simulink model "MORUS_NELINEARNI_NELINEARNI_YAW"  (R2019a)
settings: Solver=FixedStepAuto  StartTime=0.0  StopTime=sim_time  RelTol=1e-3  EnableMultiTasking=on
values from neighbouring files (symbols this model uses):
  A_dis_calc = expm(kSamplingTime*A_continous_time)    [MPC_designer_X.m]    (also in NonTilting.m; RUN_simulation.m; Simulacija_MPC_YAW_NELINEARNI.m; Simulacija_MPC_Z.m)
  A_dis_calc_YAW = expm(kSamplingTime_YAW*A_continous_time_YAW)    [Simulacija_MPC_YAW_NELINEARNI.m]
  B_dis_calc = integral_exp_A * B_continous_time    [MPC_designer_X.m]    (also in NonTilting.m; RUN_simulation.m; Simulacija_MPC_YAW_NELINEARNI.m; Simulacija_MPC_Z.m)
  B_dis_calc_YAW = integral_exp_A_YAW * B_continous_time_YAW    [Simulacija_MPC_YAW_NELINEARNI.m]
  b_f = 4.56e-4    (= 0.000456)    [LinearizacijaMatrica.m]    (also in Linearizirane_matrice.mat; MPC_designer_X.m; NonTilting.m; RUN_simulation.m)
  b_m = 0.01    [LinearizacijaMatrica.m]    (also in Linearizirane_matrice.mat; MPC_designer_X.m; NonTilting.m; RUN_simulation.m)
  BETA = 0.0    (= 0)    [LinearizacijaMatrica.m]    (also in Linearizirane_matrice.mat; MPC_designer_X.m; NonTilting.m = 0.200712863979; RUN_simulation.m)
  g = 9.80665    [LinearizacijaMatrica.m]    (also in Linearizirane_matrice.mat; MPC_designer_X.m = 9.81; NonTilting.m = 9.81; RUN_simulation.m = 9.81)
  hover = 427.6233    [MPC_designer_X.m]    (also in NonTilting.m; RUN_simulation.m; Simulacija_MPC_YAW_NELINEARNI.m; Simulacija_MPC_Z.m)
  I_b_xx = 5.5268    [MPC_designer_X.m]    (also in NonTilting.m; RUN_simulation.m; Simulacija_MPC_YAW_NELINEARNI.m; Simulacija_MPC_Z.m)
  I_b_yy = 5.5268    [MPC_designer_X.m]    (also in NonTilting.m; RUN_simulation.m; Simulacija_MPC_YAW_NELINEARNI.m; Simulacija_MPC_Z.m)
  I_b_zz = 6.8854    [MPC_designer_X.m]    (also in NonTilting.m; RUN_simulation.m; Simulacija_MPC_YAW_NELINEARNI.m; Simulacija_MPC_Z.m)
  kSamplingTime = 0.810    (= 0.81)    [MPCDesigner_YAW.m]    (also in MPC_designer_X.m = 0.1; MPC_designer_Z.m; NonTilting.m = 0.015; RUN_simulation.m = 0.015)
  kSamplingTime_YAW = 0.105    [Simulacija_MPC_YAW_NELINEARNI.m]
  L = 0.84    [LinearizacijaMatrica.m]    (also in Linearizirane_matrice.mat; MPC_designer_X.m; NonTilting.m; RUN_simulation.m)
  m = 1.0    (= 1)    [LinearizacijaMatrica.m]    (also in Linearizirane_matrice.mat; MPC_designer_X.m; NonTilting.m; RUN_simulation.m)
  M = 34.8    [LinearizacijaMatrica.m]    (also in Linearizirane_matrice.mat; MPC_designer_X.m = 34; NonTilting.m = 34; RUN_simulation.m = 34)
  m_b = 30.8    [LinearizacijaMatrica.m]    (also in Linearizirane_matrice.mat; MPC_designer_X.m; NonTilting.m; RUN_simulation.m)
  odabir = 1    [MPC_designer_X.m]    (also in NonTilting.m; RUN_simulation.m; Simulacija_MPC_YAW_NELINEARNI.m; Simulacija_MPC_Z.m)
  Q = inv(diag([0.5800 4*kSamplingTime 0.5800 4*kSamplingTime 300 300 0.2 (0.2/3) 100 4])) * diag([0, 0, 0, 0, 0, 0, 1e5,0, 1e7, 0]) *inv(diag([0.5800 4*kSamplingTime 0.5800 4*kSamplingTime 300 300 0.2 (0.2/3.0) 100 4]))    [NonTilting.m]    (also in RUN_simulation.m = diag([ 0.135340000000000,0.002706800000000,  0.1353400, 0.00; Simulacija_MPC_YAW_NELINEARNI.m = diag([pop(5),pop(6),pop(5),pop(6), pop(7),pop(7),pop(8),pop(; Simulacija_MPC_Z.m = diag([pop(5),pop(6),pop(5),pop(6), pop(7),pop(7),pop(8),pop(; Simulacija_Roll.m = diag([pop(5),pop(6),pop(5),pop(6), pop(7),pop(7),pop(8),pop()
  Q_YAW = diag([0.146606962130350,0.146606962130350,0.146606962130350,0.146606962130350,36.6517405325875,2.50697905242899])    [RUN_simulation.m]    (also in Simulacija_MPC_YAW_NELINEARNI.m = inv(diag([100 100 100 100 2*pi 1]))* diag([20 20 20 20 30000; ZaTest3.m)
  R = inv(diag([0.5800 0.5800 300 300]))*diag([0, 0, 0, 0])*inv(diag([0.5800 0.5800 300 300]))    [NonTilting.m]    (also in RUN_simulation.m = diag([0.67670, 0.67670, 0.13534000, 0.13534000]); Simulacija_MPC_YAW_NELINEARNI.m = diag([pop(1),pop(1),pop(2),pop(2)]); Simulacija_MPC_Z.m = diag([pop(1),pop(1),pop(2),pop(2)]); Simulacija_Roll.m = diag([pop(1),pop(1),pop(2),pop(2)]))
  R_delta = inv(diag([0.5800 0.5800 300 300]))* diag([0,0,0,0])*inv(diag([0.5800 0.5800 300 300]))    [NonTilting.m]    (also in RUN_simulation.m = diag([0.738879858135067, 0.738879858135067, 0.00738879858135; Simulacija_MPC_YAW_NELINEARNI.m = diag([pop(3),pop(3),pop(4),pop(4)]); Simulacija_MPC_Z.m = diag([pop(3),pop(3),pop(4),pop(4)]); Simulacija_Roll.m = diag([pop(3),pop(3),pop(4),pop(4)]))
  R_delta_YAW = diag([0,0,0,0])    [RUN_simulation.m]    (also in Simulacija_MPC_YAW_NELINEARNI.m = inv(diag([100 100 100 100]))* diag([0.1  0.1 0.1 0.1])  * in; ZaTest3.m)
  R_YAW = diag([0,0,0,0])    [RUN_simulation.m]    (also in Simulacija_MPC_YAW_NELINEARNI.m = inv(diag([100 100 100 100]))* diag([1 1 1 1])  * inv(diag([1; ZaTest3.m)
  T_r = 0.2    [LinearizacijaMatrica.m]    (also in Linearizirane_matrice.mat; MPC_designer_X.m; NonTilting.m; RUN_simulation.m)
  w_mm = 19.7845    [LinearizacijaMatrica.m]    (also in Linearizirane_matrice.mat; MPC_designer_X.m = 17; NonTilting.m = 17; RUN_simulation.m = 17)
  z_m = 0.05    [LinearizacijaMatrica.m]    (also in Linearizirane_matrice.mat; MPC_designer_X.m; NonTilting.m; RUN_simulation.m)
  z_r = 0.2    [LinearizacijaMatrica.m]    (also in Linearizirane_matrice.mat; MPC_designer_X.m; NonTilting.m; RUN_simulation.m)
  zeta_mm = 0.6544    [LinearizacijaMatrica.m]    (also in Linearizirane_matrice.mat; MPC_designer_X.m = 0.85; NonTilting.m = 0.85; RUN_simulation.m = 0.85)
libraries: simulink x8
(part 1 of 5)
settings Model: Creator=branko  LastModifiedBy=branko
settings SolverCC: AutoInsertRateTranBlk=on
settings DataIOCC: ReturnWorkspaceOutputs=off
settings DebuggingCC: ArithmeticOperatorsInVariantConditions=warning

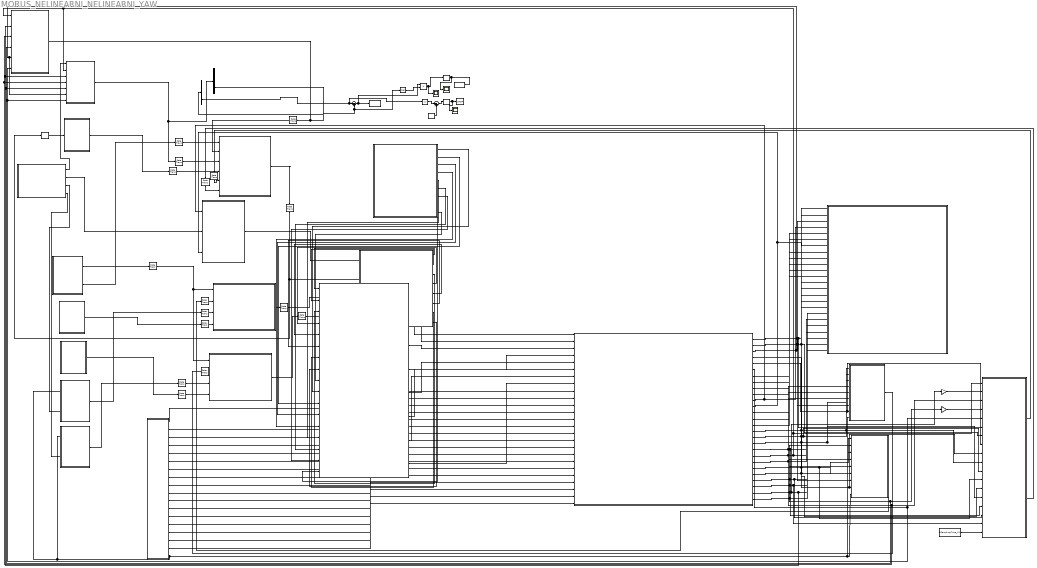
== system MORUS_NELINEARNI_NELINEARNI_YAW ==
  ACTIVATE MPC : Subsystem  Priority=1
      mask Display: image(imread('./figures/switch.PNG'))
  Abs : Abs
  Compare To Zero : simulink/Logic and Bit Operations/Compare To Zero  relop=<  OutDataTypeStr=boolean
  Compare To Zero1 : simulink/Logic and Bit Operations/Compare To Zero  relop=<  OutDataTypeStr=boolean
  Constant6 : Constant  Value=kSamplingTime_YAW
  Constant7 : Constant  Value=0.45  OutDataTypeStr=double
  DISPLAY : Subsystem  Priority=12
      mask Display: image(imread('./figures/display.png'))
  Delay : Delay  DelayLength=1
  Demux : Demux  Outputs=6
  Demux1 : Demux  Outputs=6
  Gain : Gain
  Gain1 : Gain
  KONSTANTE : Subsystem  Priority=1
      mask Display: image(imread('./figures/konst.png'))
  MANUAL REF : Subsystem  Priority=1
      mask Display: image(imread('./figures/Drone_brain.png'))
  MATLAB Function : MATLAB Function  TreatAsAtomicUnit=on  SystemSampleTime=kSamplingTime_YAW
  MORUS : Subsystem  Priority=2
      mask Display: image(imread('./figures/MORUS.png'))
  MPC PITCH : Subsystem  Priority=13
      mask Display: image(imread('./figures/Pitch1.PNG'))
  MPC ROLL : Subsystem  Priority=13
      mask Display: image(imread('./figures/Roll1.PNG'))
  PITCH SATURATION SIGNAL : Subsystem  Priority=1
      mask Display: image(imread('./figures/u_ss.PNG'))
  PITCH_SATURATION_STATE_SPACE1 : Subsystem  Priority=2
      mask Display: image(imread('./figures/x_ss.PNG'))
  PITCH_STATE_SPACE : Subsystem  Priority=12
      mask Display: image(imread('./figures/PITChss.png'))
  Product1 : Product
  REFERNCE : Subsystem  Priority=1
      mask Display: image(imread('./figures/ref.PNG'))
  REGULATOR YAW : Subsystem  Priority=13
      mask Display: image(imread('./figures/YAW1.PNG'))
  REGULATOR Z : Subsystem  Priority=13
      mask Display: image(imread('./figures/height.PNG'))
  ROLL SATURATION SIGNAL : Subsystem  Priority=1
      mask Display: image(imread('./figures/u_ss.PNG'))
  ROLL_SATURATION_STATE_SPACE : Subsystem  Priority=2
      mask Display: image(imread('./figures/x_ss.PNG'))
  ROLL_SATURATION_STATE_SPACE1 : Subsystem  Priority=2
      mask Display: image(imread('./figures/x_ss.PNG'))
  ROLL_STATE_SPACE : Subsystem  Priority=12
      mask Display: image(imread('./figures/roll_ss.png'))
  ROLL_STATE_SPACE1 : Subsystem  Priority=12
  Rate Transition{,1..8,15} (10 alike) : RateTransition  OutPortSampleTime=kSamplingTime
  Rate Transition{9..14} (6 alike) : RateTransition  OutPortSampleTime=kSamplingTime_YAW
  SIGNALS : Subsystem  Priority=4
      mask Display: image(imread('./figures/Drone_puls2.png'))
  Scope10 : Scope
  Scope12 : Scope
  Scope13 : Scope
  Sign : Signum
  Stop Simulation : Stop
  Subsystem : Subsystem  Priority=14
      mask Display: image(imread('./figures/Switch2.PNG'))
  Sum : Sum  Inputs=|-+
  Sum1 : Sum  Inputs=|-+
  To Workspace : ToWorkspace  VariableName=error_YAW  SaveFormat=Structure With Time  SampleTime=-1
  To Workspace1 : ToWorkspace  VariableName=preb_GA2  SaveFormat=Structure With Time  SampleTime=-1
  YAW SATURATION SIGNAL : Subsystem  Priority=1
      mask Display: image(imread('./figures/u_ss.PNG'))
  wires:
  KONSTANTE/1(m) -> MORUS/9(m)
  KONSTANTE/2(M) -> MORUS/10(M)
  KONSTANTE/3(L) -> MORUS/11(L)
  KONSTANTE/4(beta) -> MORUS/12(beta)
  KONSTANTE/5(b_f) -> MORUS/13(b_f)
  KONSTANTE/6(b_m) -> MORUS/14(b_m)
  KONSTANTE/7(g) -> MORUS/15(g)
  PITCH_SATURATION_STATE_SPACE1/1(PITCH_X_SS) -> Rate Transition4/1
  KONSTANTE/9(I_b_yy) -> MORUS/17(I_b_yy)
  KONSTANTE/8(I_b_xx) -> MORUS/16(I_b_xx)
  KONSTANTE/10(I_b_zz) -> MORUS/18(I_b_zz)
  KONSTANTE/11(zeta_1) -> MORUS/19(zeta_1)
  KONSTANTE/12(zeta_2) -> MORUS/20(zeta_2)
  KONSTANTE/13(zeta_3) -> MORUS/21(zeta_3)
  KONSTANTE/14(zeta_4) -> MORUS/22(zeta_4)
  KONSTANTE/15(m_b) -> MORUS/23(m_b)
  KONSTANTE/16(z_m) -> MORUS/24(z_m)
  KONSTANTE/17(z_r) -> MORUS/25(z_r)
  KONSTANTE/18(hover) -> ROLL_SATURATION_STATE_SPACE/1(hover), PITCH_SATURATION_STATE_SPACE1/1(hover), PITCH_STATE_SPACE/9(hover), ROLL_STATE_SPACE/9(hover)
  MANUAL REF/8(MANUAL_REF_ROTOR_4) -> Subsystem/17(MANUAL_REF_ROTOR_4)
  MANUAL REF/7(MANUAL_REF_ROTOR_3) -> Subsystem/16(MANUAL_REF_ROTOR_3)
  MANUAL REF/6(MANUAL_REF_ROTOR_2) -> Subsystem/15(MANUAL_REF_ROTOR_2)
  MANUAL REF/5(MANUAL_REF_ROTOR_1) -> Subsystem/14(MANUAL_REF_ROTOR_1)
  MANUAL REF/4(MANUAL_REF_MASS_4) -> Subsystem/13(MANUAL_REF_MASS_4)
  MANUAL REF/3(MANUAL_REF_MASS_3) -> Subsystem/12(MANUAL_REF_MASS_3)
  MANUAL REF/2(MANUAL_REF_MASS_2) -> Subsystem/11(MANUAL_REF_MASS_2)
  MANUAL REF/1(MANUAL_REF_MASS_1) -> Subsystem/10(MANUAL_REF_MASS_1)
  MANUAL REF/9(MANUAL_SIGNAL) -> Subsystem/9(MANUAL_SIGNAL)
  SIGNALS/1(REF_MASS_1) -> Subsystem/1(AUTO_REF_MASS_1)
  SIGNALS/2(REF_MASS_2) -> Subsystem/2(AUTO_REF_MASS_2)
  SIGNALS/3(REF_MASS_3) -> Subsystem/3(AUTO_REF_MASS_3)
  SIGNALS/4(REF_MASS_4) -> Subsystem/4(AUTO_REF_MASS_4)
  SIGNALS/5(REF_ROTOR_1) -> Subsystem/5(AUTO_REF_ROTOR_1)
  SIGNALS/6(REF_ROTOR_2) -> Subsystem/6(AUTO_REF_ROTOR_2)
  SIGNALS/7(REF_ROTOR_3) -> Subsystem/7(AUTO_REF_ROTOR_3)
  SIGNALS/8(REF_ROTOR_4) -> Subsystem/8(AUTO_REF_ROTOR_4)
  MPC PITCH/1(SIGNAL_PITCH) -> Rate Transition8/1
  PITCH SATURATION SIGNAL/1(PITCH_SATURATION_SIGNAL) -> Rate Transition5/1
  ACTIVATE MPC/1(KRENI) -> Rate Transition/1
  PITCH_STATE_SPACE/1(PITCH_STATE_SPACE) -> MPC PITCH/2(PITCH_STATE_SPACE)
  ROLL_SATURATION_STATE_SPACE/1(ROLL_X_SS) -> Rate Transition2/1
  REFERNCE/3(REF_ROLL) -> ROLL_SATURATION_STATE_SPACE/2(REF_ROLL)
  REFERNCE/4(REF_PITCH) -> PITCH_SATURATION_STATE_SPACE1/2(REF_PITCH)
  MPC ROLL/1(SIGNAL_ROLL) -> Rate Transition7/1
  ROLL SATURATION SIGNAL/1(ROLL_SATURATION_SIGNAL) -> Rate Transition3/1
  ROLL_STATE_SPACE/1(ROLL_STATE_SPACE) -> Rate Transition1/1
  MORUS/12(DOT_Z) -> REGULATOR Z/3(DOT_Z), DISPLAY/7(DOT_Z)
  REFERNCE/2(REF_Z) -> REGULATOR Z/2(REF_Z)
  REGULATOR Z/1(SIGNAL_Z) -> SIGNALS/1(SIGNAL_Z)
  MORUS/3(YAW) -> DISPLAY/3(YAW), ROLL_SATURATION_STATE_SPACE1/6(5), ROLL_STATE_SPACE1/5(YAW)
  MORUS/11(Z) -> REGULATOR Z/1(Z), DISPLAY/4(Z)
  REGULATOR YAW/1(SIGNAL_YAW) -> Rate Transition15/1
  MORUS/1(ROLL) -> DISPLAY/1(ROLL), MATLAB Function/6(ROLL), ROLL_STATE_SPACE/7(ROLL)
  MORUS/2(PITCH) -> DISPLAY/2(PITCH), MATLAB Function/7(PITCH), PITCH_STATE_SPACE/7(PITCH)
  MORUS/7(X) -> DISPLAY/5(X)
  MORUS/9(Y) -> DISPLAY/6(Y)
  MORUS/8(DOT_X) -> DISPLAY/8(DOT_X)
  MORUS/10(DOT_Y) -> DISPLAY/9(DOT_Y)
  MORUS/13(DOT_DOT_Z) -> DISPLAY/10(DOT_DOT_Z)
  MORUS/15(DOT_DOT_X) -> DISPLAY/11(DOT_DOT_X)
  MORUS/14(DOT_DOT_Y) -> DISPLAY/12(DOT_DOT_Y)
  MORUS/16(x_1) -> PITCH_STATE_SPACE/1(x_1), MATLAB Function/10(x_1), DISPLAY/13(masa_x_1)
  MORUS/22(y_2) -> ROLL_STATE_SPACE/1(y_2), MATLAB Function/12(y_2), DISPLAY/14(masa_y_2)
  MORUS/17(x_3) -> PITCH_STATE_SPACE/3(x_3), MATLAB Function/11(x_3), DISPLAY/15(masa_x_3)
  MORUS/4(DOT_ROLL) -> MATLAB Function/9(DOT_ROLL), ROLL_STATE_SPACE/8(DOT_ROLL)
  MORUS/5(DOT_PITCH) -> MATLAB Function/8(DOT_PITCH), PITCH_STATE_SPACE/8(DOT_PITCH)
  MORUS/18(DOT_x_1) -> PITCH_STATE_SPACE/2(DOT_x_1), MATLAB Function/14(DOT_x_1), DISPLAY/17(DOT_masa_x_1)
  MORUS/23(y_4) -> ROLL_STATE_SPACE/3(y_4), DISPLAY/16(masa_y_4), MATLAB Function/13(y_4)
  MORUS/24(DOT_y_2) -> DISPLAY/18(DOT_masa_y_2), MATLAB Function/16(DOT_y_2), ROLL_STATE_SPACE/2(DOT_y_2)
  MORUS/27(ROTOR_4) -> ROLL_SATURATION_STATE_SPACE1/5(4), ROLL_STATE_SPACE1/4(ROTOR_4), Gain1/1, DISPLAY/24(ROTOR_4), ROLL_STATE_SPACE/6(ROTOR_4)
  MORUS/21(ROTOR_3) -> ROLL_SATURATION_STATE_SPACE1/4(3), ROLL_STATE_SPACE1/3(ROTOR_3), MATLAB Function/3(OMEGA_3), DISPLAY/23(ROTOR_3), PITCH_STATE_SPACE/6(ROTOR_3)
  MORUS/26(ROTOR_2) -> DISPLAY/22(ROTOR_2), ROLL_SATURATION_STATE_SPACE1/3(2), ROLL_STATE_SPACE1/2(ROTOR_2), Gain/1, ROLL_STATE_SPACE/5(ROTOR_2)
  MORUS/20(ROTOR_1) -> MATLAB Function/1(OMEGA_1), ROLL_SATURATION_STATE_SPACE1/2(1), ROLL_STATE_SPACE1/1(ROTOR_1), DISPLAY/21(ROTOR_1), PITCH_STATE_SPACE/5(ROTOR_1)
  MORUS/25(DOT_y_4) -> DISPLAY/20(DOT_masa_y_4), MATLAB Function/17(DOT_y_4), ROLL_STATE_SPACE/4(DOT_y_4)
  MORUS/19(DOT_x_3) -> DISPLAY/19(DOT_masa_x_3), MATLAB Function/15(DOT_x_3), PITCH_STATE_SPACE/4(DOT_x_3)
  Subsystem/1(REF_MASS_1) -> MORUS/1(ref_masa_1)
  Subsystem/2(REF_MASS_2) -> MORUS/2(ref_masa_2)
  Subsystem/3(REF_MASS_3) -> MORUS/3(ref_masa_3)
  Subsystem/4(REF_MASS_4) -> MORUS/4(ref_masa_4)
  Subsystem/5(REF_ROTOR_1) -> MORUS/5(ref_rotor_1)
  Subsystem/6(REF_ROTOR_2) -> MORUS/6(ref_rotor_2)
  Subsystem/7(REF_ROTOR_3) -> MORUS/7(ref_rotor_3)
  Subsystem/8(REF_ROTOR_4) -> MORUS/8(ref_rotor_4)
  YAW SATURATION SIGNAL/1(YAW_SATURATION_SIGNAL) -> Rate Transition11/1
  REFERNCE/1(REF_YAW) -> ROLL_SATURATION_STATE_SPACE1/1(REF_YAW)
  ACTIVATE MPC/2(KRENI_yaw) -> Rate Transition9/1
  MORUS/6(DOT_YAW) -> ROLL_SATURATION_STATE_SPACE1/7(6), ROLL_STATE_SPACE1/6(DOT_YAW), MATLAB Function/5(DOT_YAW)
  ROLL_STATE_SPACE1/1(YAW_STATE_SPACE) -> Demux/1, Rate Transition14/1
  MATLAB Function/1(A_dis_calc) -> Rate Transition13/1
  MATLAB Function/2(B_dis_calc) -> Rate Transition12/1
  Constant6/1 -> MATLAB Function/18(kSamplingTime)
  Gain/1 -> MATLAB Function/2(OMEGA_2)
  Gain1/1 -> MATLAB Function/4(OMEGA_4)
  Rate Transition/1 -> MPC PITCH/1(KRENI), MPC ROLL/1(KRENI)
  Rate Transition1/1 -> MPC ROLL/2(ROLL_STATE_SPACE)
  Rate Transition2/1 -> MPC ROLL/3(ROLL_SATURATION_STATE_SPACE)
  Rate Transition3/1 -> MPC ROLL/4(ROLL_SIGNAL_SATURATION)
  Rate Transition4/1 -> MPC PITCH/3(PITCH_SATURATION_STATE_SPACE)
  Rate Transition5/1 -> MPC PITCH/4(PITCH_SIGNAL_SATURATION)
  Rate Transition7/1 -> SIGNALS/3(SIGNAL_ROLL)
  Rate Transition8/1 -> SIGNALS/4(SIGNAL_PITCH)
  Rate Transition9/1 -> REGULATOR YAW/1(KRENI)
  Rate Transition10/1 -> REGULATOR YAW/3(YAW_SATURATION_STATE_SPACE)
  Rate Transition11/1 -> REGULATOR YAW/4(YAW_SIGNAL_SATURATION)
  Rate Transition12/1 -> REGULATOR YAW/6(B)
  Rate Transition13/1 -> REGULATOR YAW/5(A)
  Rate Transition14/1 -> REGULATOR YAW/2(YAW_STATE_SPACE)
  Rate Transition15/1 -> Delay/1, SIGNALS/2(SIGNAL_YAW)
  Demux1/5 -> Sum/2, Sign/1
  Sum1/1 -> Compare To Zero/1
  Sign/1 -> Product1/2
  Compare To Zero/1 -> Scope10/1, Stop Simulation/1
  Product1/1 -> Scope13/1, Compare To Zero1/1
  Abs/1 -> Sum1/1
  Constant7/1 -> Sum1/2
  Demux/5 -> Abs/1, Sum/1
  Compare To Zero1/1 -> Scope12/1, To Workspace1/1
  Sum/1 -> To Workspace/1, Product1/1
  ROLL_SATURATION_STATE_SPACE1/1(YAW_X_SS) -> Demux1/1, Rate Transition10/1
  Delay/1 -> YAW SATURATION SIGNAL/1(1)

== system MORUS_NELINEARNI_NELINEARNI_YAW/ACTIVATE MPC ==
  Clock : Clock
  Clock1 : Clock
  Constant1 : Constant  OutDataTypeStr=double  SampleTime=-1
  Constant2 : Constant  Value=0  OutDataTypeStr=double  SampleTime=-1
  Constant3 : Constant  Value=10  OutDataTypeStr=double  SampleTime=-1
  Constant6 : Constant  OutDataTypeStr=double  SampleTime=-1
  Constant7 : Constant  Value=0  OutDataTypeStr=double  SampleTime=-1
  Constant8 : Constant  Value=5  OutDataTypeStr=double  SampleTime=-1
  Sum1 : Sum  Inputs=|+-
  Sum9 : Sum  Inputs=|+-
  Switch : Switch  Criteria=u2 > Threshold
  Switch1 : Switch  Criteria=u2 > Threshold
  KRENI : Outport
  KRENI_yaw : Outport  Port=2
  wires:
  Constant6/1 -> Switch/1
  Clock/1 -> Sum9/1
  Constant8/1 -> Sum9/2
  Sum9/1 -> Switch/2  "Error"
  Constant7/1 -> Switch/3
  Switch/1 -> KRENI/1
  Constant3/1 -> Sum1/2
  Constant2/1 -> Switch1/3
  Switch1/1 -> KRENI_yaw/1
  Sum1/1 -> Switch1/2  "Error"
  Clock1/1 -> Sum1/1
  Constant1/1 -> Switch1/1

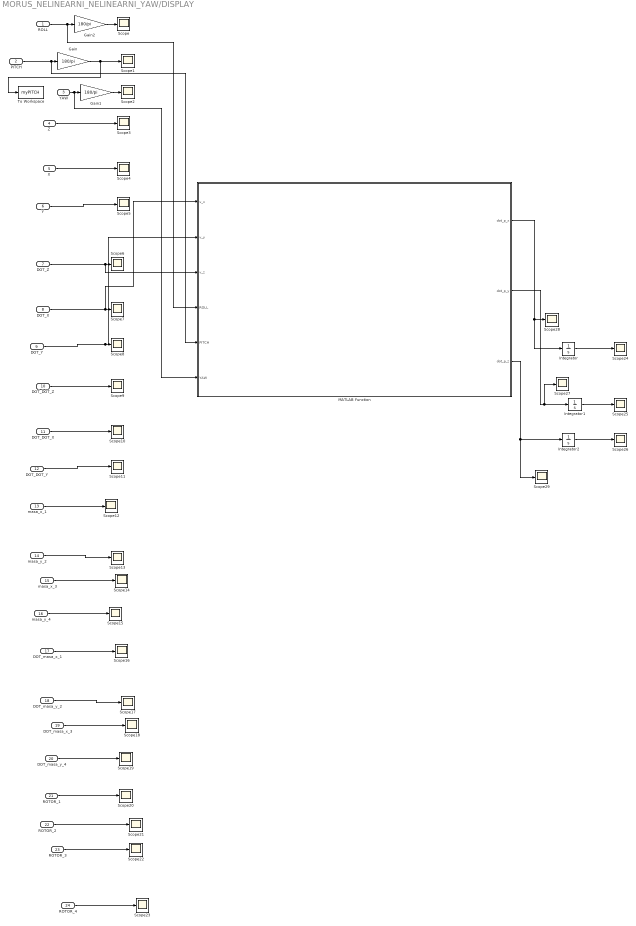
== system MORUS_NELINEARNI_NELINEARNI_YAW/DISPLAY ==
  ROLL : Inport
  PITCH : Inport  Port=2
  YAW : Inport  Port=3
  Z : Inport  Port=4
  X : Inport  Port=5
  Y : Inport  Port=6
  DOT_Z : Inport  Port=7
  DOT_X : Inport  Port=8
  DOT_Y : Inport  Port=9
  DOT_DOT_Z : Inport  Port=10
  DOT_DOT_X : Inport  Port=11
  DOT_DOT_Y : Inport  Port=12
  masa_x_1 : Inport  Port=13
  masa_y_2 : Inport  Port=14
  masa_x_3 : Inport  Port=15
  masa_y_4 : Inport  Port=16
  DOT_masa_x_1 : Inport  Port=17
  DOT_masa_y_2 : Inport  Port=18
  DOT_masa_x_3 : Inport  Port=19
  DOT_masa_y_4 : Inport  Port=20
  ROTOR_1 : Inport  Port=21
  ROTOR_2 : Inport  Port=22
  ROTOR_3 : Inport  Port=23
  ROTOR_4 : Inport  Port=24
  Gain : Gain  Gain=180/pi
  Gain1 : Gain  Gain=180/pi
  Gain2 : Gain  Gain=180/pi
  Integrator : Integrator
  Integrator1 : Integrator
  Integrator2 : Integrator
  MATLAB Function : MATLAB Function  TreatAsAtomicUnit=on
  Scope{,1..29} (30 alike) : Scope
  To Workspace : ToWorkspace  VariableName=myPITCH  SaveFormat=Structure With Time  SampleTime=-1
  wires:
  ROLL/1 -> MATLAB Function/4(ROLL), Gain2/1
  PITCH/1 -> MATLAB Function/5(PITCH), Gain/1
  YAW/1 -> MATLAB Function/6(YAW), Gain1/1
  Z/1 -> Scope3/1
  Gain/1 -> To Workspace/1, Scope1/1
  Gain1/1 -> Scope2/1
  Gain2/1 -> Scope/1
  X/1 -> Scope4/1
  Y/1 -> Scope5/1
  DOT_X/1 -> MATLAB Function/1(v_x), Scope7/1
  DOT_Y/1 -> MATLAB Function/2(v_y), Scope8/1
  DOT_Z/1 -> MATLAB Function/3(v_z), Scope6/1
  DOT_DOT_Y/1 -> Scope11/1
  DOT_DOT_X/1 -> Scope10/1
  DOT_DOT_Z/1 -> Scope9/1
  masa_x_1/1 -> Scope12/1
  masa_y_2/1 -> Scope13/1
  masa_x_3/1 -> Scope14/1
  masa_y_4/1 -> Scope15/1
  DOT_masa_y_2/1 -> Scope17/1
  DOT_masa_y_4/1 -> Scope19/1
  DOT_masa_x_1/1 -> Scope16/1
  DOT_masa_x_3/1 -> Scope18/1
  ROTOR_1/1 -> Scope20/1
  ROTOR_2/1 -> Scope21/1
  ROTOR_3/1 -> Scope22/1
  ROTOR_4/1 -> Scope23/1
  Integrator2/1 -> Scope26/1
  Integrator1/1 -> Scope25/1
  MATLAB Function/2(dot_p_y) -> Scope27/1, Integrator1/1
  MATLAB Function/3(dot_p_z) -> Scope29/1, Integrator2/1
  Integrator/1 -> Scope24/1
  MATLAB Function/1(dot_p_x) -> Integrator/1, Scope28/1

== system MORUS_NELINEARNI_NELINEARNI_YAW/KONSTANTE ==
  Constant : Constant  Value=m  OutDataTypeStr=double  SampleTime=-1
  Constant1 : Constant  Value=M  OutDataTypeStr=double  SampleTime=-1
  Constant{10..13} (4 alike) : Constant  OutDataTypeStr=double  SampleTime=-1
  Constant14 : Constant  Value=m_b  OutDataTypeStr=double  SampleTime=-1
  Constant15 : Constant  Value=z_m  OutDataTypeStr=double  SampleTime=-1
  Constant16 : Constant  Value=z_r  OutDataTypeStr=double  SampleTime=-1
  Constant17 : Constant  Value=hover  OutDataTypeStr=double  SampleTime=-1
  Constant2 : Constant  Value=L  OutDataTypeStr=double  SampleTime=-1
  Constant3 : Constant  Value=BETA  OutDataTypeStr=double  SampleTime=-1
  Constant4 : Constant  Value=b_f  OutDataTypeStr=double  SampleTime=-1
  Constant5 : Constant  Value=b_m  OutDataTypeStr=double  SampleTime=-1
  Constant6 : Constant  Value=g  OutDataTypeStr=double  SampleTime=-1
  Constant7 : Constant  Value=I_b_xx  OutDataTypeStr=double  SampleTime=-1
  Constant8 : Constant  Value=I_b_yy  OutDataTypeStr=double  SampleTime=-1
  Constant9 : Constant  Value=I_b_zz  OutDataTypeStr=double  SampleTime=-1
  m : Outport
  M : Outport  Port=2
  L : Outport  Port=3
  beta : Outport  Port=4
  b_f : Outport  Port=5
  b_m : Outport  Port=6
  g : Outport  Port=7
  I_b_xx : Outport  Port=8
  I_b_yy : Outport  Port=9
  I_b_zz : Outport  Port=10
  zeta_1 : Outport  Port=11
  zeta_2 : Outport  Port=12
  zeta_3 : Outport  Port=13
  zeta_4 : Outport  Port=14
  m_b : Outport  Port=15
  z_m : Outport  Port=16
  z_r : Outport  Port=17
  hover : Outport  Port=18
  wires:
  Constant/1 -> m/1
  Constant3/1 -> beta/1
  Constant2/1 -> L/1
  Constant1/1 -> M/1
  Constant4/1 -> b_f/1
  Constant5/1 -> b_m/1
  Constant6/1 -> g/1
  Constant7/1 -> I_b_xx/1
  Constant8/1 -> I_b_yy/1
  Constant9/1 -> I_b_zz/1
  Constant10/1 -> zeta_1/1
  Constant11/1 -> zeta_2/1
  Constant12/1 -> zeta_3/1
  Constant13/1 -> zeta_4/1
  Constant14/1 -> m_b/1
  Constant15/1 -> z_m/1
  Constant16/1 -> z_r/1
  Constant17/1 -> hover/1

== system MORUS_NELINEARNI_NELINEARNI_YAW/MANUAL REF ==
  Abs{,1..7} (8 alike) : Abs
  Add : Sum  Inputs=++++++++
  Constant{,1..3,9} (5 alike) : Constant  Value=0  OutDataTypeStr=double
  Constant4 : Constant  Value=400  OutDataTypeStr=double
  Constant5 : Constant  Value=420  OutDataTypeStr=double
  Constant6 : Constant  Value=400  OutDataTypeStr=double
  Constant7 : Constant  Value=420  OutDataTypeStr=double
  Constant8 : Constant  OutDataTypeStr=double
  Manual Switch : ManualSwitch  CurrentSetting=0
  Product{,1..7} (8 alike) : Product
  MANUAL_REF_MASS_1 : Outport
  MANUAL_REF_MASS_2 : Outport  Port=2
  MANUAL_REF_MASS_3 : Outport  Port=3
  MANUAL_REF_MASS_4 : Outport  Port=4
  MANUAL_REF_ROTOR_1 : Outport  Port=5
  MANUAL_REF_ROTOR_2 : Outport  Port=6
  MANUAL_REF_ROTOR_3 : Outport  Port=7
  MANUAL_REF_ROTOR_4 : Outport  Port=8
  MANUAL_SIGNAL : Outport  Port=9
  wires:
  Product/1 -> Abs/1, MANUAL_REF_MASS_1/1
  Product1/1 -> Abs1/1, MANUAL_REF_MASS_2/1
  Product2/1 -> Abs2/1, MANUAL_REF_MASS_3/1
  Product3/1 -> MANUAL_REF_MASS_4/1, Abs3/1
  Product4/1 -> MANUAL_REF_ROTOR_1/1, Abs4/1
  Product5/1 -> MANUAL_REF_ROTOR_2/1, Abs5/1
  Product6/1 -> MANUAL_REF_ROTOR_3/1, Abs6/1
  Product7/1 -> MANUAL_REF_ROTOR_4/1, Abs7/1
  Add/1 -> MANUAL_SIGNAL/1
  Abs/1 -> Add/1
  Abs1/1 -> Add/2
  Abs2/1 -> Add/3
  Abs3/1 -> Add/4
  Abs4/1 -> Add/5
  Abs5/1 -> Add/6
  Abs6/1 -> Add/7
  Abs7/1 -> Add/8
  Constant/1 -> Product/2
  Constant8/1 -> Manual Switch/1
  Constant9/1 -> Manual Switch/2
  Manual Switch/1 -> [MANUAL]
  [MANUAL] -> Product/1
  [MANUAL] -> Product1/1
  Constant1/1 -> Product1/2
  [MANUAL] -> Product2/1
  Constant2/1 -> Product2/2
  [MANUAL] -> Product3/1
  Constant3/1 -> Product3/2
  [MANUAL] -> Product4/1
  Constant4/1 -> Product4/2
  [MANUAL] -> Product5/1
  Constant5/1 -> Product5/2
  [MANUAL] -> Product6/1
  Constant6/1 -> Product6/2
  [MANUAL] -> Product7/1
  Constant7/1 -> Product7/2

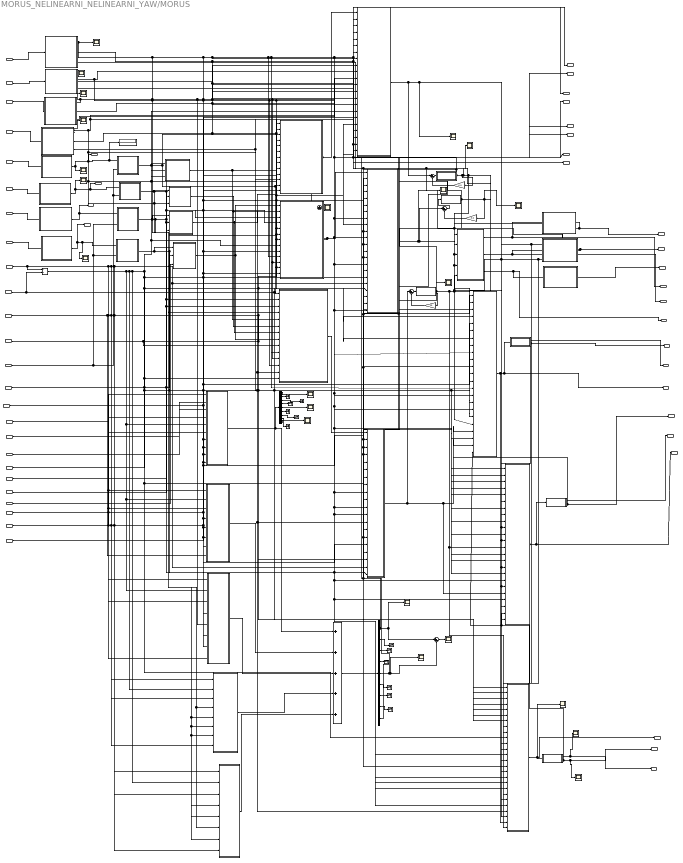
== system MORUS_NELINEARNI_NELINEARNI_YAW/MORUS ==
  ref_masa_1 : Inport
  ref_masa_2 : Inport  Port=2
  ref_masa_3 : Inport  Port=3
  ref_masa_4 : Inport  Port=4
  ref_rotor_1 : Inport  Port=5
  ref_rotor_2 : Inport  Port=6
  ref_rotor_3 : Inport  Port=7
  ref_rotor_4 : Inport  Port=8
  m : Inport  Port=9
  M : Inport  Port=10
  L : Inport  Port=11
  beta : Inport  Port=12
  b_f : Inport  Port=13
  b_m : Inport  Port=14
  g : Inport  Port=15
  I_b_xx : Inport  Port=16
  I_b_yy : Inport  Port=17
  I_b_zz : Inport  Port=18
  zeta_1 : Inport  Port=19
  zeta_2 : Inport  Port=20
  zeta_3 : Inport  Port=21
  zeta_4 : Inport  Port=22
  m_b : Inport  Port=23
  z_m : Inport  Port=24
  z_r : Inport  Port=25
  DOT_V_X : Subsystem  Priority=10
  DOT_V_Y : Subsystem  Priority=10
  DOT_V_Z : Subsystem  Priority=10
  Demux : Demux  Outputs=9
  Demux1 : Demux  Outputs=9
  Display : Display
      settings: Decimation=5
  Divide : Product  Priority=2  Inputs=*/  OutDataTypeStr=double
  Force rotor 1 : Subsystem  Priority=3
      mask Display: image(imread('f1.png'))
  Force rotor 2 : Subsystem  Priority=3
      mask Display: image(imread('f2.png'))
  Force rotor 3 : Subsystem  Priority=3
      mask Display: image(imread('f3.png'))
  Force rotor 4 : Subsystem  Priority=3
      mask Display: image(imread('f4.png'))
  Gain : Gain  Gain=5.0
  Gain1 : Gain  Gain=5.0
  Gain2 : Gain  Gain=10
  ICE ROTOR 2 : Subsystem  Priority=2
      mask Display: image(imread('rotor.PNG'))
  ICE ROTOR 3 : Subsystem  Priority=2
      mask Display: image(imread('rotor.PNG'))
  ICE ROTOR 4 : Subsystem  Priority=2
      mask Display: image(imread('rotor.PNG'))
  ICE(Internal combustion engine) ROTOR 1 : Subsystem  Priority=2
      mask Display: image(imread('rotor.PNG'))
  I_1_c : Subsystem  Priority=3
  I_2_c : Subsystem  Priority=3
  I_3_c : Subsystem  Priority=3
  I_4_c : Subsystem  Priority=3
  I_b_c : Subsystem  Priority=3
  I_s_c : Sum  Priority=4  Inputs=+++++  AccumDataTypeStr=double  OutDataTypeStr=double
  MATLAB Function : MATLAB Function  Priority=8  TreatAsAtomicUnit=on
  M_e_x : Subsystem  Priority=5
      mask Display: image(imread('mx.png'))
  M_e_y : Subsystem  Priority=5
      mask Display: image(imread('my.png'))
  M_e_z : Subsystem  Priority=5
      mask Display: image(imread('mz.png'))
  Moment rotor 1 : Subsystem  Priority=4
      mask Display: image(imread('m1.png'))
  Moment rotor 2 : Subsystem  Priority=4
      mask Display: image(imread('m2.png'))
  Moment rotor 3 : Subsystem  Priority=4
      mask Display: image(imread('m3.png'))
  Moment rotor 4 : Subsystem  Priority=4
      mask Display: image(imread('m4.png'))
  SERVO MASA 1 : Subsystem  Priority=2  TreatAsAtomicUnit=on
      mask Display: image(imread('Mass.PNG'))
  SERVO MASA 2 : Subsystem  Priority=2  TreatAsAtomicUnit=on
      mask Display: image(imread('Mass.PNG'))
  SERVO MASA 3 : Subsystem  Priority=2  TreatAsAtomicUnit=on
      mask Display: image(imread('Mass.PNG'))
  SERVO MASA 4 : Subsystem  Priority=2  TreatAsAtomicUnit=on
      mask Display: image(imread('Mass.PNG'))
  Scope{,1..21} (22 alike) : Scope
  Subsystem1 : Subsystem  Priority=7
  Subsystem2 : Subsystem  Priority=7
  Subsystem3 : Subsystem  Priority=7
  Subsystem4 : Subsystem  Priority=9
      mask Display: image(imread('Roll1.png'))
  Subsystem5 : Subsystem  Priority=9
      mask Display: image(imread('Pitch1.png'))
  Subsystem6 : Subsystem  Priority=9
      mask Display: image(imread('Yaw1.png'))
  Subsystem7 : Subsystem  Priority=11
  Subsystem8 : Subsystem  Priority=11
  Subsystem9 : Subsystem  Priority=11
  Sum{,1..4} (5 alike) : Sum  Inputs=|+-
  Terminator{,1..11} (12 alike) : Terminator
  dot_w_x : Subsystem  Priority=6
  dot_w_y : Subsystem  Priority=6
  dot_w_z : Subsystem  Priority=6
  ROLL : Outport
  PITCH : Outport  Port=2
  YAW : Outport  Port=3
  DOT_ROLL : Outport  Port=4
  DOT_PITCH : Outport  Port=5
  DOT_YAW : Outport  Port=6
  X : Outport  Port=7
  DOT_X : Outport  Port=8
  Y : Outport  Port=9
  DOT_Y : Outport  Port=10
  Z : Outport  Port=11
  DOT_Z : Outport  Port=12
  DOT_DOT_Z : Outport  Port=13
  DOT_DOT_Y : Outport  Port=14
  DOT_DOT_X : Outport  Port=15
  x_1 : Outport  Port=16
  x_3 : Outport  Port=17
  DOT_x_1 : Outport  Port=18
  DOT_x_3 : Outport  Port=19
  ROTOR_1 : Outport  Port=20
  ROTOR_3 : Outport  Port=21
  y_2 : Outport  Port=22
  y_4 : Outport  Port=23
  DOT_y_2 : Outport  Port=24
  DOT_y_4 : Outport  Port=25
  ROTOR_2 : Outport  Port=26
  ROTOR_4 : Outport  Port=27
  wires:
  ref_masa_4/1 -> SERVO MASA 4/1(ref_masa_4)
  ref_masa_3/1 -> SERVO MASA 3/1(ref_masa_3)
  ref_masa_2/1 -> SERVO MASA 2/1(ref_masa_2)
  ref_masa_1/1 -> SERVO MASA 1/1(ref_masa_1)
  ref_rotor_1/1 -> ICE(Internal combustion engine) ROTOR 1/1(ref_rotor_1)
  ref_rotor_2/1 -> ICE ROTOR 2/1(ref_rotor_2)
  ref_rotor_3/1 -> ICE ROTOR 3/1(ref_rotor_3)
  ref_rotor_4/1 -> ICE ROTOR 4/1(ref_rotor_4)
  ICE(Internal combustion engine) ROTOR 1/1(rotor_1) -> ROTOR_1/1, Display/1, Force rotor 1/1(rotor_1), Scope16/1
  ICE ROTOR 2/1(rotor_2) -> Scope17/1, ROTOR_2/1, Force rotor 2/1(rotor_2)
  ICE ROTOR 3/1(rotor_3) -> ROTOR_3/1, Force rotor 3/1(rotor_3)
  ICE ROTOR 4/1(rotor_4) -> ROTOR_4/1, Scope12/1, Force rotor 4/1(rotor_4)
  m/1 -> I_1_c/1(m), I_2_c/1(m), dot_w_y/18(m), dot_w_z/19(m), dot_w_x/18(m), I_4_c/1(m), I_3_c/1(m), Divide/1
  M/1 -> DOT_V_Y/1(M), DOT_V_Z/1(M), DOT_V_X/1(M), Divide/2
  I_1_c/1(I_1_c) -> I_s_c/2
  I_2_c/1(I_2_c) -> I_s_c/3
  I_3_c/1(I_3_c) -> I_s_c/4
  I_4_c/1(I_4_c) -> I_s_c/5
  DOT_V_X/1(DOT_V_X) -> Subsystem8/1("DOT_DOT_X "), DOT_DOT_X/1, DOT_V_Z/25(V_0_X)
  DOT_V_Y/1(DOT_V_Y) -> Subsystem7/1("DOT_DOT_Y "), DOT_DOT_Y/1, DOT_V_Z/26(V_0_Y)
  DOT_V_Z/1(DOT_V_Z) -> DOT_DOT_Z/1, Subsystem9/1("DOT_DOT_Z "), Scope3/1
  SERVO MASA 1/1(masa_1/x1) -> I_3_c/6(x1), I_4_c/4(x_1), I_1_c/6(x1), I_2_c/4(x1), I_b_c/9(x1), DOT_V_Y/17(X_1), DOT_V_Z/18(X_1), dot_w_y/10(x_1), dot_w_z/8(x_1), x_1/1, M_e_z/10(x1), DOT_V_X/14(X_1), M_e_y/10(x1), dot_w_x/8(x1), Scope8/1
  SERVO MASA 2/1(masa_2/y2) -> I_3_c/4(y2), I_4_c/6(y2), I_1_c/4(y2), I_2_c/6(y_2), I_b_c/7(y2), DOT_V_Z/22(Y_2), dot_w_z/12(y_2), DOT_V_Y/14(Y_2_), DOT_V_X/17(Y_2), dot_w_y/8(y2), y_2/1, M_e_x/10(y2), M_e_z/12(y2), dot_w_x/10(y2), Scope9/1
  SERVO MASA 3/1(masa_3/x3) -> Scope10/1, I_3_c/7(x3), I_4_c/5(x_3), I_b_c/10(x3), I_1_c/7(x3), M_e_z/11(x3), M_e_y/11(x3), DOT_V_Y/18(X_3), DOT_V_Z/19(X_3), dot_w_z/9(x_3), DOT_V_X/15(X_3), dot_w_y/11(x_3), x_3/1, dot_w_x/9(x3), I_2_c/5(x3)
  SERVO MASA 4/1(masa_4/y4) -> I_3_c/5(y4), I_4_c/7(y4), I_1_c/5(y4), I_2_c/7(y4), I_b_c/8(y4), DOT_V_Z/23(Y_4), dot_w_z/13(y_4), DOT_V_X/18(Y_4), DOT_V_Y/15(Y_4_), M_e_z/13(y4), dot_w_y/9(y4), M_e_x/11(y4), dot_w_x/11(y4), y_4/1, Scope11/1
  I_s_c/1 -> Demux/1  "errors"
  Demux/1 -> dot_w_y/2(I_s_c_xx_), dot_w_z/4(I_s_c_xx), dot_w_x/3(I_s_c_xx), Scope18/1, Sum3/1
  Demux/5 -> dot_w_y/3(I_s_c_yy_), dot_w_z/3(I_s_c_yy), dot_w_x/4(I_s_c_yy), Scope19/1, Sum3/2
  M_e_x/1(M_e_x) -> Sum4/1, dot_w_x/1(M_e_x)
  M_e_y/1(M_e_y) -> Sum4/2, dot_w_y/1(M_e_y)
  Subsystem1/1(W_X) -> MATLAB Function/3(W_X), DOT_V_X/16(W_X), DOT_V_Y/12(W_X_), DOT_V_Z/16(W_X), Scope13/1, Gain/1, dot_w_x/5(w_x), dot_w_y/6(w_x_), dot_w_z/5(w_x)
  Subsystem3/1(W_Z) -> dot_w_y/7(w_z), dot_w_z/7(w_z), DOT_V_Y/13(W_Z), DOT_V_Z/20(W_Z), MATLAB Function/5(W_Z), DOT_V_X/13(W_Z), Scope15/1, Gain2/1, dot_w_x/7(w_z)
  Subsystem9/2(DOT_Z) -> Scope5/1, DOT_Z/1, DOT_V_X/23(V_0_Z), DOT_V_Y/23(V_0_Z)
  Subsystem9/1(Z) -> Scope4/1, Z/1
  I_b_c/1(I_b_c) -> Demux1/1, I_s_c/1
  Demux1/1 -> Scope/1
  Demux1/9 -> Scope1/1
  Demux1/5 -> Scope2/1
  Sum/1 -> Subsystem1/1("DOT_W_X ")  "Error"
  Gain/1 -> Sum/2
  Gain1/1 -> Sum1/2
  Subsystem2/1(W_Y) -> MATLAB Function/4(W_Y), DOT_V_X/12(W_Y), dot_w_z/6(w_y), DOT_V_Y/16(W_Y_), DOT_V_Z/11(W_Y), Scope14/1, Gain1/1, dot_w_x/6(w_y), dot_w_y/5(w_y_)
  Sum1/1 -> Subsystem2/1("DOT_W_Y ")  "Error"
  Sum2/1 -> Subsystem3/1("DOT_W_Z ")  "Error"
  Gain2/1 -> Sum2/2
  Sum3/1 -> Scope20/1
  Sum4/1 -> Scope21/1
  Demux/2 -> Terminator1/1
  Demux/3 -> Terminator/1
  Demux/4 -> Terminator2/1
  Demux/6 -> Terminator3/1
  Demux/7 -> Terminator4/1
  Demux/8 -> Terminator5/1
  Demux1/2 -> Terminator6/1
  Demux1/3 -> Terminator7/1
  Demux1/4 -> Terminator8/1
  Demux1/6 -> Terminator9/1
  Demux1/7 -> Terminator10/1
  Demux1/8 -> Terminator11/1
  I_b_xx/1 -> I_b_c/1(I_b_xx)
  I_b_yy/1 -> I_b_c/2(I_b_yy)
  I_b_zz/1 -> I_b_c/3(I_b_zz)
  z_m/1 -> DOT_V_Y/21(z_m), DOT_V_Z/17(z_m), dot_w_z/20(z_m), dot_w_x/20(z_m), M_e_x/9(z_m), M_e_y/9(z_m), dot_w_y/20(z_m), DOT_V_X/21(z_m), I_4_c/3(z_m), I_3_c/3(z_m), I_b_c/6(z_m), I_1_c/3(z_m), I_2_c/3(z_m)
  m_b/1 -> dot_w_x/17(m_b), dot_w_y/17(m_b), dot_w_z/16(m_b), I_b_c/4(m_b)
  Divide/1 -> I_1_c/2(mi), I_2_c/2(mi), I_b_c/5(mi), DOT_V_Z/10(mi), dot_w_z/17(mi), DOT_V_Y/7(mi), M_e_z/14(mi), DOT_V_X/7(mi), dot_w_y/16(mi), dot_w_x/16(mi), M_e_x/8(mi), M_e_y/8(mi), I_4_c/2(mi), I_3_c/2(mi)
  g/1 -> DOT_V_X/5(g), DOT_V_Y/5(g), DOT_V_Z/7(g)
  b_m/1 -> Moment rotor 3/2(b_m), Moment rotor 2/2(b_m), Moment rotor 4/2(b_m), Moment rotor 1/2(b_m)
  b_f/1 -> Force rotor 1/2(b_f), Force rotor 2/2(b_f), Force rotor 3/2(b_f), Force rotor 4/2(b_f)
  beta/1 -> DOT_V_Y/4(BETA), DOT_V_Z/6(BETA), M_e_x/7(BETA), M_e_y/7(BETA), DOT_V_X/4(BETA), M_e_z/9(BETA)
  L/1 -> dot_w_x/19(L), M_e_x/12(L), M_e_y/12(L), dot_w_y/19(L), dot_w_z/18(L), I_4_c/8(L), I_3_c/8(L), I_2_c/8(L), I_1_c/8(L)
  zeta_1/1 -> Moment rotor 1/3(zeta_1)
  SERVO MASA 1/2("dot_x_1 ") -> dot_w_y/14(dot_x_1), dot_w_z/10(dot_x_1), DOT_V_Y/10(DOT_X_1_), DOT_V_Z/12(DOT_X_1), DOT_x_1/1, dot_w_x/12(dot_x1)
  SERVO MASA 1/3("dot_dot_x_1 ") -> DOT_V_X/8(DOT_DOT_X_1), dot_w_y/21(dot_dot_x1)
  SERVO MASA 2/2("dot_y_2 ") -> dot_w_y/12(dot_y2), dot_w_z/14(dot_y_2), DOT_V_X/10(DOT_Y_2), DOT_V_Z/14(DOT_Y_2), DOT_y_2/1, dot_w_x/14(dot_y2)
  SERVO MASA 2/3("dot_dot_y_2 ") -> DOT_V_Y/8(DOT_DOT_Y_2), dot_w_x/21(dot_dot_y2)
  SERVO MASA 3/2("dot_x_3 ") -> DOT_V_Z/13(DOT_X_3), dot_w_z/11(dot_x_3), DOT_V_Y/11(DOT_X_3_), dot_w_y/15(dot_x_3), DOT_x_3/1, dot_w_x/13(dot_x3)
  SERVO MASA 3/3("dot_dot_x_3 ") -> DOT_V_X/9(DOT_DOT_X_3), dot_w_y/22(dot_dot_x3)
  Demux/9 -> dot_w_y/4(I_s_c_zz_), dot_w_z/2(I_s_c_zz), dot_w_x/2(I_s_c_zz)
  Moment rotor 1/1(Moment_1) -> M_e_x/1(M_r_1), M_e_z/5(M_r_1)
  Moment rotor 3/1(Moment_3) -> M_e_x/2(M_r_3), M_e_z/7(M_r_3)
  Force rotor 1/1(Force_1) -> DOT_V_X/3(F_r_1), DOT_V_Z/2(F_r_1), M_e_y/6(F_r1), M_e_z/1(F_r_1), M_e_x/3(F_r_1), Moment rotor 1/1(Force_1)
  SERVO MASA 4/2("dot_y_4 ") -> DOT_V_Z/15(DOT_Y_4), dot_w_z/15(dot_y_4), DOT_V_X/11(DOT_Y_4), dot_w_y/13(dot_y4), DOT_y_4/1, dot_w_x/15(dot_y4)
  SERVO MASA 4/3("dot_dot_y_4 ") -> dot_w_x/22(dot_dot_y4), DOT_V_Y/9(DOT_DOT_Y_4)
  Force rotor 2/1(Force_2) -> DOT_V_Z/3(F_r_2), M_e_z/2(F_r_2), M_e_y/3(F_r2), M_e_x/4(F_r_2), DOT_V_Y/3(F_r_2), Moment rotor 2/1(Force_2)
  Force rotor 3/1(Force_3) -> DOT_V_Z/4(F_r_3), M_e_z/3(F_r_3), M_e_x/5(F_r_3), M_e_y/4(F_r3), DOT_V_X/2(F_r_3), Moment rotor 3/1(Force_3)
  Force rotor 4/1(Force_4) -> DOT_V_Y/2(F_r_4), DOT_V_Z/5(F_r_4), M_e_z/4(F_r_4), M_e_x/6(F_r_4), M_e_y/5(F_r4), Moment rotor 4/1(Force_4)
  zeta_3/1 -> Moment rotor 3/3(zeta_3)
  zeta_2/1 -> Moment rotor 2/3(zeta_2)
  Moment rotor 2/1(Moment_2) -> M_e_y/2(M_r_2), M_e_z/6(M_r_2)
  z_r/1 -> M_e_x/13(z_r), M_e_y/13(z_r)
  Moment rotor 4/1(Moment_4) -> M_e_y/1(M_r_4), M_e_z/8(M_r_4)
  zeta_4/1 -> Moment rotor 4/3(zeta_4)
  M_e_z/1(M_e_z) -> dot_w_z/1(M_e_z)
  dot_w_z/1(dot_w_z) -> DOT_V_X/20(DOT_W_Z), DOT_V_Y/20(DOT_W_Z), Sum2/1
  Subsystem5/1(PITCH) -> DOT_V_X/6(PITCH), DOT_V_Y/6(PITCH), DOT_V_Z/9(PITCH), MATLAB Function/2(PITCH), PITCH/1
  MATLAB Function/2(DOT_PITCH) -> DOT_PITCH/1, Subsystem5/1("DOT_PITCH ")
  MATLAB Function/1(DOT_ROLL) -> DOT_ROLL/1, Subsystem4/1("DOT_ROLL ")
  dot_w_y/1(dot_w_y) -> DOT_V_X/19(DOT_W_Y), DOT_V_Z/21(DOT_W_Y), Sum1/1, Scope7/1
  Subsystem8/1(X) -> X/1
  Subsystem8/2(DOT_X) -> DOT_V_Y/22(V_0_X), DOT_X/1
  MATLAB Function/3(DOT_YAW) -> DOT_YAW/1, Subsystem6/1("DOT_YAW ")
  dot_w_x/1(dot_w_x) -> DOT_V_Y/19(DOT_W_X), DOT_V_Z/24(DOT_W_X), Scope6/1, Sum/1
  Subsystem4/1(ROLL) -> DOT_V_Y/24(ROLL), DOT_V_Z/8(ROLL), MATLAB Function/1(ROLL), ROLL/1
  Subsystem6/1(YAW) -> YAW/1
  Subsystem7/2(DOT_Y) -> DOT_V_X/22(V_0_Y), DOT_Y/1
  Subsystem7/1(Y) -> Y/1

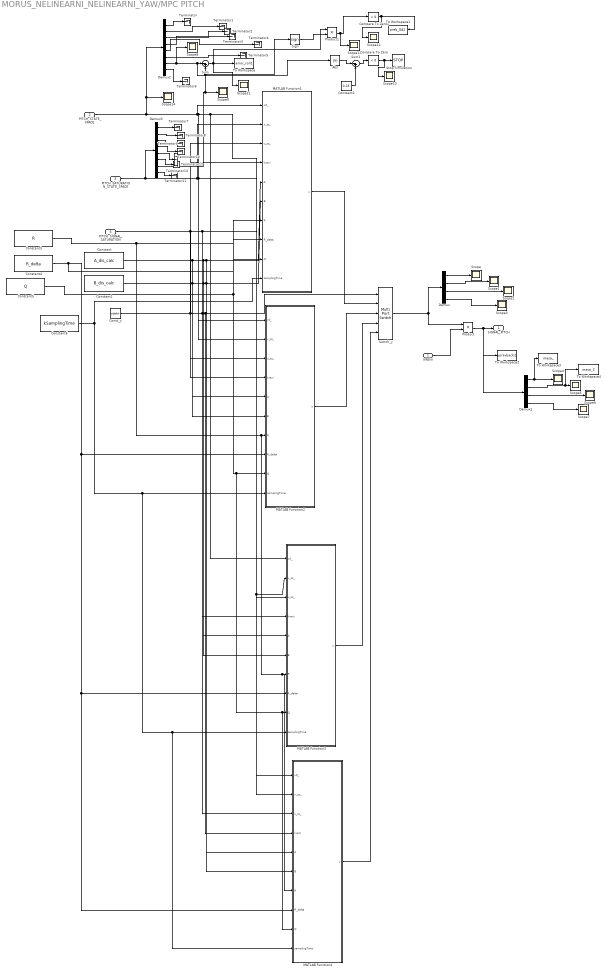
== system MORUS_NELINEARNI_NELINEARNI_YAW/MPC PITCH ==
  KRENI : Inport
  PITCH_STATE_SPACE : Inport  Port=2
  PITCH_SATURATION_STATE_SPACE : Inport  Port=3
  PITCH_SIGNAL_SATURATION : Inport  Port=4
  Abs : Abs
  Compare To Zero : simulink/Logic and Bit Operations/Compare To Zero  relop=<  OutDataTypeStr=boolean
  Compare To Zero1 : simulink/Logic and Bit Operations/Compare To Zero  relop=<  OutDataTypeStr=boolean
  Const_y : Constant  Value=odabir
  Constant : Constant  Value=A_dis_calc
  Constant1 : Constant  Value=B_dis_calc
  Constant2 : Constant  Value=0.25  OutDataTypeStr=double
  Constant3 : Constant  Value=R
  Constant4 : Constant  Value=R_delta
  Constant5 : Constant  Value=Q
  Constant6 : Constant  Value=kSamplingTime
  Demux : Demux
  Demux1 : Demux
  Demux2 : Demux  Outputs=8
  Demux3 : Demux  Outputs=8
  MATLAB Function1 : MATLAB Function  TreatAsAtomicUnit=on  SystemSampleTime=kSamplingTime
  MATLAB Function2 : MATLAB Function  TreatAsAtomicUnit=on  SystemSampleTime=kSamplingTime
  MATLAB Function3 : MATLAB Function  TreatAsAtomicUnit=on  SystemSampleTime=kSamplingTime
  MATLAB Function4 : MATLAB Function  TreatAsAtomicUnit=on  SystemSampleTime=kSamplingTime
  Product : Product
  Product1 : Product
  Scope{,1..14} (15 alike) : Scope
  Sign : Signum
  Stop Simulation : Stop
  Sum : Sum  Inputs=|-+
  Sum1 : Sum  Inputs=|-+
  Switch_y : MultiPortSwitch  Inputs=4  DiagnosticForDefault=None
  Terminator{,1..13} (14 alike) : Terminator
  To Workspace : ToWorkspace  VariableName=error_roll1  SaveFormat=Structure With Time  SampleTime=-1
  To Workspace1 : ToWorkspace  VariableName=preb_GA1  SaveFormat=Structure With Time  SampleTime=-1
  To Workspace2 : ToWorkspace  VariableName=upravljacki1  SaveFormat=Structure With Time  SampleTime=kSamplingTime
  To Workspace3 : ToWorkspace  VariableName=masa_  SaveFormat=Structure With Time  SampleTime=-1
  To Workspace4 : ToWorkspace  VariableName=masa_3  SaveFormat=Structure With Time  SampleTime=-1
  SIGNAL_PITCH : Outport
  wires:
  PITCH_SATURATION_STATE_SPACE/1 -> Demux3/1, MATLAB Function3/2(x_ss_), MATLAB Function4/2(x_ss_), MATLAB Function2/2(x_ss_), MATLAB Function1/2(x_ss_)
  PITCH_SIGNAL_SATURATION/1 -> MATLAB Function3/3(u_ss_), MATLAB Function4/3(u_ss_), MATLAB Function1/3(u_ss_), MATLAB Function2/3(u_ss_)
  Const_y/1 -> Switch_y/1, MATLAB Function4/4(kreni), MATLAB Function3/4(kreni), MATLAB Function1/4(kreni), MATLAB Function2/4(kreni)
  Constant/1 -> MATLAB Function1/5(A), MATLAB Function4/5(A), MATLAB Function3/5(A), MATLAB Function2/5(A)
  Demux3/7 -> Sum/2, Sign/1, Scope9/1
  Demux1/3 -> Scope6/1
  Demux2/8 -> Terminator6/1
  Constant1/1 -> MATLAB Function1/6(B), MATLAB Function4/6(B), MATLAB Function3/6(B), MATLAB Function2/6(B)
  Compare To Zero/1 -> Scope10/1, Stop Simulation/1
  Demux/1 -> Scope/1
  Sum1/1 -> Compare To Zero/1
  Demux2/7 -> Scope8/1, Abs/1, Sum/1
  Demux3/5 -> Terminator13/1
  Switch_y/1 -> Demux/1, Product/1
  MATLAB Function2/1(u) -> Switch_y/3
  MATLAB Function3/1(u) -> Switch_y/4
  MATLAB Function4/1(u) -> Switch_y/5
  Constant6/1 -> MATLAB Function4/10(samplingTime), MATLAB Function3/10(samplingTime), MATLAB Function2/10(samplingTime), MATLAB Function1/10(samplingTime)
  KRENI/1 -> Product/2
  MATLAB Function1/1(u) -> Switch_y/2
  Abs/1 -> Sum1/1
  Compare To Zero1/1 -> Scope12/1, To Workspace1/1
  Demux3/3 -> Terminator9/1
  Demux1/1 -> To Workspace3/1, Scope4/1
  Constant5/1 -> MATLAB Function4/9(Q), MATLAB Function3/9(Q), MATLAB Function2/9(Q), MATLAB Function1/9(Q)
  Sum/1 -> Scope11/1, To Workspace/1, Product1/1
  Product/1 -> To Workspace2/1, SIGNAL_PITCH/1, Demux1/1
  Demux2/2 -> Terminator1/1
  Demux3/2 -> Terminator8/1
  PITCH_STATE_SPACE/1 -> Scope14/1, Demux2/1, MATLAB Function3/1(x0_), MATLAB Function4/1(x0_), MATLAB Function2/1(x0_), MATLAB Function1/1(x0_)
  Demux3/1 -> Terminator7/1
  Demux2/4 -> Terminator3/1
  Demux3/8 -> Terminator11/1
  Demux1/2 -> To Workspace4/1, Scope5/1
  Product1/1 -> Scope13/1, Compare To Zero1/1
  Demux2/1 -> Terminator/1
  Demux3/6 -> Terminator12/1
  Demux1/4 -> Scope7/1
  Demux2/3 -> Terminator2/1
  Demux/3 -> Scope2/1
  Demux/4 -> Scope3/1
  Sign/1 -> Product1/2
  Demux2/6 -> Terminator5/1
  Constant3/1 -> MATLAB Function4/7(R), MATLAB Function3/7(R), MATLAB Function2/7(R), MATLAB Function1/7(R)
  Constant2/1 -> Sum1/2
  Demux/2 -> Scope1/1
  Demux2/5 -> Terminator4/1
  Constant4/1 -> MATLAB Function2/8(R_delta), MATLAB Function3/8(R_delta), MATLAB Function4/8(R_delta), MATLAB Function1/8(R_delta)
  Demux3/4 -> Terminator10/1

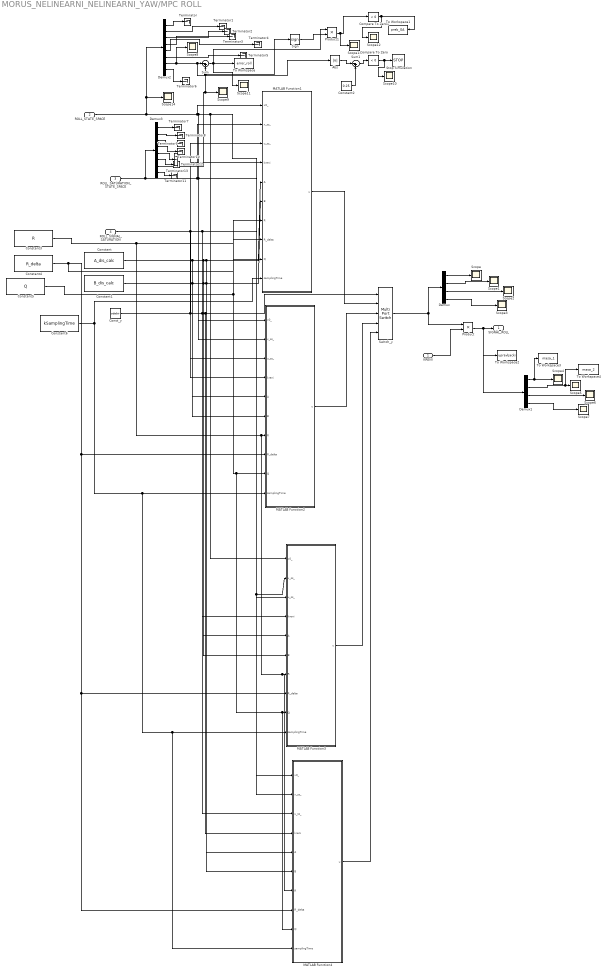
== system MORUS_NELINEARNI_NELINEARNI_YAW/MPC ROLL ==
  KRENI : Inport
  ROLL_STATE_SPACE : Inport  Port=2
  ROLL_SATURATION_STATE_SPACE : Inport  Port=3
  ROLL_SIGNAL_SATURATION : Inport  Port=4
  Abs : Abs
  Compare To Zero : simulink/Logic and Bit Operations/Compare To Zero  relop=<  OutDataTypeStr=boolean
  Compare To Zero1 : simulink/Logic and Bit Operations/Compare To Zero  relop=<  OutDataTypeStr=boolean
  Const_y : Constant  Value=odabir
  Constant : Constant  Value=A_dis_calc
  Constant1 : Constant  Value=B_dis_calc
  Constant2 : Constant  Value=0.25  OutDataTypeStr=double
  Constant3 : Constant  Value=R
  Constant4 : Constant  Value=R_delta
  Constant5 : Constant  Value=Q
  Constant6 : Constant  Value=kSamplingTime
  Demux : Demux
  Demux1 : Demux
  Demux2 : Demux  Outputs=8
  Demux3 : Demux  Outputs=8
  MATLAB Function1 : MATLAB Function  TreatAsAtomicUnit=on  SystemSampleTime=kSamplingTime
  MATLAB Function2 : MATLAB Function  TreatAsAtomicUnit=on  SystemSampleTime=kSamplingTime
  MATLAB Function3 : MATLAB Function  TreatAsAtomicUnit=on  SystemSampleTime=kSamplingTime
  MATLAB Function4 : MATLAB Function  TreatAsAtomicUnit=on  SystemSampleTime=kSamplingTime
  Product : Product
  Product1 : Product
  Scope{,1..14} (15 alike) : Scope
  Sign : Signum
  Stop Simulation : Stop
  Sum : Sum  Inputs=|-+
  Sum1 : Sum  Inputs=|-+
  Switch_y : MultiPortSwitch  Inputs=4  DiagnosticForDefault=None
  Terminator{,1..13} (14 alike) : Terminator
  To Workspace : ToWorkspace  VariableName=error_roll  SaveFormat=Structure With Time  SampleTime=-1
  To Workspace1 : ToWorkspace  VariableName=preb_GA  SaveFormat=Structure With Time  SampleTime=-1
  To Workspace2 : ToWorkspace  VariableName=upravljacki  SaveFormat=Structure With Time  SampleTime=kSamplingTime
  To Workspace3 : ToWorkspace  VariableName=masa_1  SaveFormat=Structure With Time  SampleTime=-1
  To Workspace4 : ToWorkspace  VariableName=masa_2  SaveFormat=Structure With Time  SampleTime=-1
  SIGNAL_ROLL : Outport
  wires:
  KRENI/1 -> Product/2
  Demux/1 -> Scope/1
  Demux/2 -> Scope1/1
  Demux/3 -> Scope2/1
  Demux/4 -> Scope3/1
  Demux1/1 -> To Workspace3/1, Scope4/1
  Product/1 -> To Workspace2/1, SIGNAL_ROLL/1, Demux1/1
  Demux1/4 -> Scope7/1
  Demux1/3 -> Scope6/1
  Demux1/2 -> To Workspace4/1, Scope5/1
  MATLAB Function1/1(u) -> Switch_y/2
  MATLAB Function2/1(u) -> Switch_y/3
  MATLAB Function3/1(u) -> Switch_y/4
  MATLAB Function4/1(u) -> Switch_y/5
  ROLL_STATE_SPACE/1 -> Scope14/1, Demux2/1, MATLAB Function3/1(x0_), MATLAB Function4/1(x0_), MATLAB Function2/1(x0_), MATLAB Function1/1(x0_)
  ROLL_SATURATION_STATE_SPACE/1 -> Demux3/1, MATLAB Function3/2(x_ss_), MATLAB Function4/2(x_ss_), MATLAB Function2/2(x_ss_), MATLAB Function1/2(x_ss_)
  ROLL_SIGNAL_SATURATION/1 -> MATLAB Function3/3(u_ss_), MATLAB Function4/3(u_ss_), MATLAB Function1/3(u_ss_), MATLAB Function2/3(u_ss_)
  Constant/1 -> MATLAB Function1/5(A), MATLAB Function4/5(A), MATLAB Function3/5(A), MATLAB Function2/5(A)
  Constant1/1 -> MATLAB Function1/6(B), MATLAB Function4/6(B), MATLAB Function3/6(B), MATLAB Function2/6(B)
  Const_y/1 -> Switch_y/1, MATLAB Function4/4(kreni), MATLAB Function3/4(kreni), MATLAB Function1/4(kreni), MATLAB Function2/4(kreni)
  Demux2/7 -> Scope8/1, Abs/1, Sum/1
  Demux3/7 -> Sum/2, Sign/1, Scope9/1
  Sum/1 -> Scope11/1, To Workspace/1, Product1/1
  Demux2/1 -> Terminator/1
  Demux2/2 -> Terminator1/1
  Demux2/3 -> Terminator2/1
  Demux2/4 -> Terminator3/1
  Demux2/5 -> Terminator4/1
  Demux2/6 -> Terminator5/1
  Demux2/8 -> Terminator6/1
  Demux3/1 -> Terminator7/1
  Demux3/2 -> Terminator8/1
  Demux3/3 -> Terminator9/1
  Demux3/4 -> Terminator10/1
  Demux3/8 -> Terminator11/1
  Demux3/6 -> Terminator12/1
  Demux3/5 -> Terminator13/1
  Compare To Zero/1 -> Scope10/1, Stop Simulation/1
  Abs/1 -> Sum1/1
  Sum1/1 -> Compare To Zero/1
  Constant2/1 -> Sum1/2
  Constant3/1 -> MATLAB Function4/7(R), MATLAB Function3/7(R), MATLAB Function2/7(R), MATLAB Function1/7(R)
  Constant4/1 -> MATLAB Function2/8(R_delta), MATLAB Function3/8(R_delta), MATLAB Function4/8(R_delta), MATLAB Function1/8(R_delta)
  Constant5/1 -> MATLAB Function4/9(Q), MATLAB Function3/9(Q), MATLAB Function2/9(Q), MATLAB Function1/9(Q)
  Sign/1 -> Product1/2
  Product1/1 -> Scope13/1, Compare To Zero1/1
  Compare To Zero1/1 -> Scope12/1, To Workspace1/1
  Switch_y/1 -> Demux/1, Product/1
  Constant6/1 -> MATLAB Function4/10(samplingTime), MATLAB Function3/10(samplingTime), MATLAB Function2/10(samplingTime), MATLAB Function1/10(samplingTime)

== system MORUS_NELINEARNI_NELINEARNI_YAW/PITCH SATURATION SIGNAL ==
  Constant : Constant  Value=0  OutDataTypeStr=double  SampleTime=-1
  Mux2 : Mux
  PITCH_SATURATION_SIGNAL : Outport
  wires:
  Constant/1 -> Mux2/1, Mux2/4, Mux2/3, Mux2/2
  Mux2/1 -> PITCH_SATURATION_SIGNAL/1  "PropSpeedCmd"

== system MORUS_NELINEARNI_NELINEARNI_YAW/PITCH_SATURATION_STATE_SPACE1 ==
  hover : Inport
  REF_PITCH : Inport  Port=2
  Constant : Constant  Value=0  OutDataTypeStr=double  SampleTime=-1
  Mux2 : Mux  Inputs=8
  PITCH_X_SS : Outport
  wires:
  Mux2/1 -> PITCH_X_SS/1  "PropSpeedCmd"
  Constant/1 -> Mux2/3, Mux2/6, Mux2/5, Mux2/8, Mux2/4, Mux2/1, Mux2/2
  REF_PITCH/1 -> Mux2/7

== system MORUS_NELINEARNI_NELINEARNI_YAW/PITCH_STATE_SPACE ==
  x_1 : Inport
  DOT_x_1 : Inport  Port=2
  x_3 : Inport  Port=3
  DOT_x_3 : Inport  Port=4
  ROTOR_1 : Inport  Port=5
  ROTOR_3 : Inport  Port=6
  PITCH : Inport  Port=7
  DOT_PITCH : Inport  Port=8
  hover : Inport  Port=9
  Display : Display
      settings: Decimation=5
  Mux : Mux  Inputs=8
  Scope : Scope
  Sum : Sum  Inputs=|+-
  Sum1 : Sum  Inputs=|+-
  PITCH_STATE_SPACE : Outport
  wires:
  Mux/1 -> PITCH_STATE_SPACE/1
  x_1/1 -> Mux/1
  DOT_x_1/1 -> Mux/2
  x_3/1 -> Mux/3
  DOT_x_3/1 -> Mux/4
  PITCH/1 -> Mux/7
  DOT_PITCH/1 -> Mux/8
  ROTOR_1/1 -> Sum/1
  ROTOR_3/1 -> Display/1, Scope/1, Sum1/1
  Sum1/1 -> Mux/5
  Sum/1 -> Mux/6
  hover/1 -> Sum/2, Sum1/2

== system MORUS_NELINEARNI_NELINEARNI_YAW/REFERNCE ==
  Constant : Constant  Value=12*(pi/180)  OutDataTypeStr=double
  Constant1 : Constant  Value=0*(pi/180)  OutDataTypeStr=double
  Constant2 : Constant  Value=5.0  OutDataTypeStr=double
  Constant3 : Constant  Value=0*(pi/180)  OutDataTypeStr=double
  Product : Product
  Product1 : Product
  Scope : Scope
  Step : Step  Time=20  SampleTime=0
  Step1 : Step  Time=50  After=2  SampleTime=0
  Step2 : Step  Time=100  After=2  SampleTime=0
  Step3 : Step  Time=10  SampleTime=0
  Sum : Sum  Inputs=|+-+
  Terminator1 : Terminator
  REF_YAW : Outport
  REF_Z : Outport  Port=2
  REF_ROLL : Outport  Port=3
  REF_PITCH : Outport  Port=4
  wires:
  Product1/1 -> REF_YAW/1
  Constant2/1 -> REF_Z/1
  Constant1/1 -> Product/1
  Step1/1 -> Sum/2
  Step/1 -> Sum/1
  Sum/1 -> Product/2
  Constant3/1 -> Terminator1/1
  Step2/1 -> Sum/3
  Product/1 -> REF_ROLL/1, REF_PITCH/1, Scope/1
  Constant/1 -> Product1/1
  Step3/1 -> Product1/2

== system MORUS_NELINEARNI_NELINEARNI_YAW/REGULATOR YAW ==
  KRENI : Inport
  YAW_STATE_SPACE : Inport  Port=2
  YAW_SATURATION_STATE_SPACE : Inport  Port=3
  YAW_SIGNAL_SATURATION : Inport  Port=4
  A : Inport  Port=5
  B : Inport  Port=6
  Constant1 : Constant  Value=A_dis_calc_YAW
  Constant2 : Constant  Value=B_dis_calc_YAW
  Constant3 : Constant  Value=R_YAW
  Constant4 : Constant  Value=R_delta_YAW
  Constant5 : Constant  Value=Q_YAW
  Constant6 : Constant  Value=kSamplingTime_YAW
  Demux : Demux
  Demux1 : Demux  Outputs=6
  Demux2 : Demux  Outputs=6
  Display : Display
  Display1 : Display
  Display2 : Display
  MATLAB Function1 : MATLAB Function  TreatAsAtomicUnit=on  SystemSampleTime=kSamplingTime_YAW
  Product : Product
  Scope{,1..6} (7 alike) : Scope
  Terminator{,1..3} (4 alike) : Terminator
  SIGNAL_YAW : Outport
  wires:
  YAW_SIGNAL_SATURATION/1 -> MATLAB Function1/3(u_ss_)
  Demux/3 -> Scope2/1
  Product/1 -> SIGNAL_YAW/1
  Constant6/1 -> MATLAB Function1/9(samplingTime)
  B/1 -> Terminator1/1
  KRENI/1 -> MATLAB Function1/10(kreni), Product/2
  Constant4/1 -> MATLAB Function1/7(R_delta)
  Demux/4 -> Scope3/1
  Demux/2 -> Scope1/1
  Demux/1 -> Scope/1
  Constant5/1 -> MATLAB Function1/8(Q)
  A/1 -> Terminator/1
  Constant3/1 -> MATLAB Function1/6(R)
  Constant1/1 -> MATLAB Function1/4(A), Terminator2/1
  Constant2/1 -> MATLAB Function1/5(B), Terminator3/1
  Demux1/1 -> Scope4/1
  Demux1/5 -> Scope5/1
  Demux1/6 -> Scope6/1
  Demux2/1 -> Display/1
  Demux2/6 -> Display2/1
  MATLAB Function1/1(u) -> Product/1, Demux/1
  YAW_SATURATION_STATE_SPACE/1 -> Demux2/1, MATLAB Function1/2(x_ss_)
  YAW_STATE_SPACE/1 -> Demux1/1, MATLAB Function1/1(x0_)
  ? -> ?
  Demux2/5 -> Display1/1
